simulink library "drf"  (Simulink 8.1)
settings: Solver=ode1  StartTime=0.0  StopTime=Inf  FixedStep=0.001  RelTol=1e-3
PostLoadFcn:
  | , if any(exist('dsrtsu_mdlpostloadfcn', 'file') == [2, 3, 6]), try dsrtsu_mdlpostloadfcn('Execute', bdroot); catch fprintf('Error in PostLoadFcn (dsrtsu_mdlpostloadfcn) for model "%s":\n %s\n', bdroot, lasterr); end, end,
undefined symbols (not defined in the file or in its folder): ZERO_FLOAT
libraries: drd x1, drg x1
settings Model: DSRTSU_INTERNAL_RTI_VER=450  DSRTSU_INTERNAL_RTI_TYPE=rti1401  RTICANMMDATA=struct('GeneralSetupData',struct('modelroot','D:\ELN150201_TAIWAN\trunk\AdasDragon\software\sw_development\arch\app\acc','generalsettings',struct('filesettings',struct('destfolder',struct('Name','RTICANMM_FILES','Check',1),'buildfolder',struct('Name','.','Check',1),'AbsDestfolder',struct('Name','D:\ELN150201_TAIWAN\trunk\AdasDragon\software\sw_development\arch\app\acc\RTICANMM_FILES'),'AbsBuildfolder',struct('Name','D:\ELN150201_TAIWAN\trunk\AdasDragon\software\sw_development\arch\app\acc'))),'options',struct('addpaths',1,'rmpaths',1,'addtrcexclusion',logical(1),'cannavigator',struct('checkmonitoring',0),'show_usrtrc',0,'use_usrtrc',0),'advanced',struct('options',[1 1 1 1 1 1 1 1 1 1 1 1 1 1 1 1 1 1 1 1 1 1 1 1 1 1 1 1 1 1 1 1 1 1 1 1 1 1 1 1 1 1 1 1 1 1 1 1 1 1 1 1 1 1 1 1 1 1 1 1 1 1 1 1 1 1 1 1 1 1 1 1 1 1 1 1 1 1 1 1 1 1 1 1 1 1 1 1 1 1 1 1 1 1 1 1 1 1 1 1]),'MPSetup',{{}},'modelname','drd','block','drd'))  DSRTSU_INTERNAL_RTIFPGA=40  Creator=AT015555  LastModifiedBy=AT015555

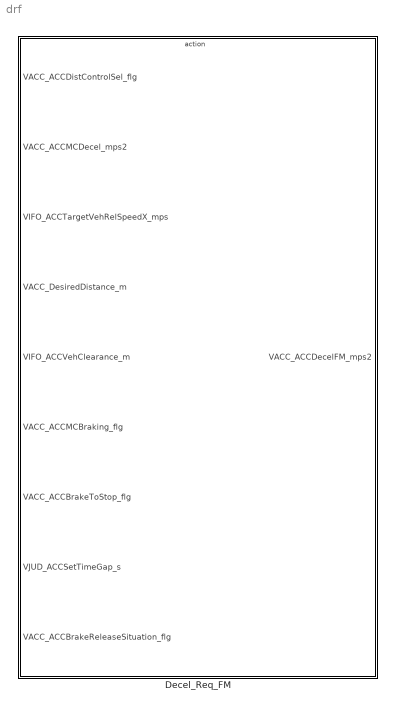
== system drf ==
  Decel_Req_FM : Subsystem  TreatAsAtomicUnit=on

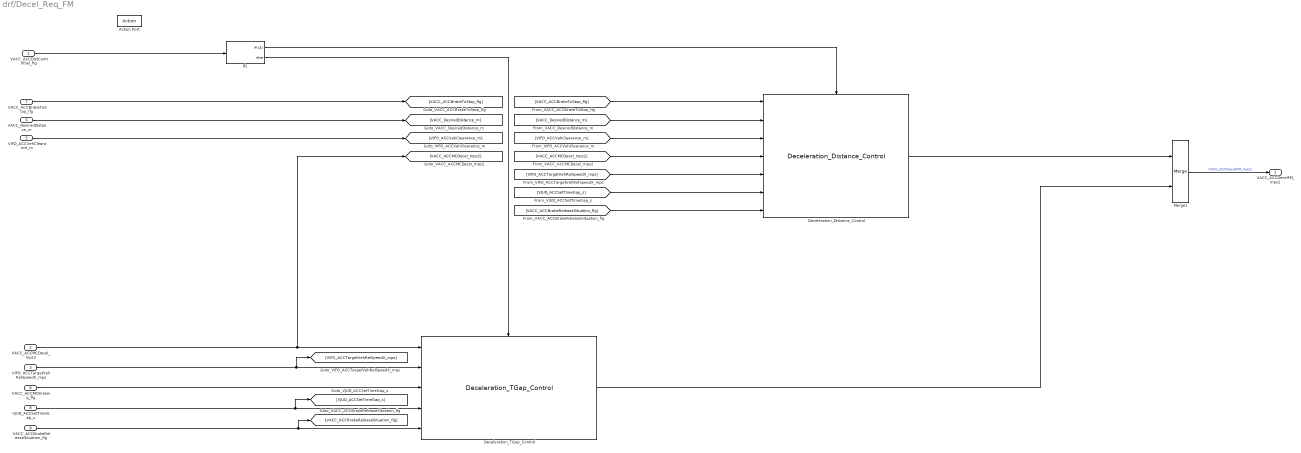
== system drf/Decel_Req_FM ==
  VACC_ACCDistControlSel_flg : Inport
  VACC_ACCMCDecel_mps2 : Inport  Port=2
  VIFO_ACCTargetVehRelSpeedX_mps : Inport  Port=3
  VACC_DesiredDistance_m : Inport  Port=4
  VIFO_ACCVehClearance_m : Inport  Port=5
  VACC_ACCMCBraking_flg : Inport  Port=6
  VACC_ACCBrakeToStop_flg : Inport  Port=7
  VJUD_ACCSetTimeGap_s : Inport  Port=8
  VACC_ACCBrakeReleaseSituation_flg : Inport  Port=9
  Action Port : ActionPort
  Deceleration_Distance_Control : drd/Deceleration_Distance_Control
  Deceleration_TGap_Control : drg/Deceleration_TGap_Control
  If2 : If  IfExpression=u1
  Merge1 : Merge
  VACC_ACCDecelFM_mps2 : Outport  OutputWhenDisabled=reset  InitialOutput=ZERO_FLOAT
  wires:
  VACC_ACCDistControlSel_flg/1 -> If2/1
  VACC_ACCMCDecel_mps2/1 -> Deceleration_TGap_Control/1, [VACC_ACCMCDecel_mps2]
  Merge1/1 -> VACC_ACCDecelFM_mps2/1  "VACC_ACCDecelFM_mps2"
  If2/2 -> Deceleration_TGap_Control/Action
  If2/1 -> Deceleration_Distance_Control/Action
  VIFO_ACCTargetVehRelSpeedX_mps/1 -> Deceleration_TGap_Control/2, [VIFO_ACCTargetVehRelSpeedX_mps]
  VACC_DesiredDistance_m/1 -> [VACC_DesiredDistance_m]
  [VACC_DesiredDistance_m] -> Deceleration_Distance_Control/2
  VIFO_ACCVehClearance_m/1 -> [VIFO_ACCVehClearance_m]
  [VIFO_ACCVehClearance_m] -> Deceleration_Distance_Control/3
  Deceleration_Distance_Control/1 -> Merge1/1
  Deceleration_TGap_Control/1 -> Merge1/2
  VACC_ACCMCBraking_flg/1 -> Deceleration_TGap_Control/3
  [VIFO_ACCTargetVehRelSpeedX_mps] -> Deceleration_Distance_Control/5
  [VACC_ACCMCDecel_mps2] -> Deceleration_Distance_Control/4
  VACC_ACCBrakeToStop_flg/1 -> [VACC_ACCBrakeToStop_flg]
  [VACC_ACCBrakeToStop_flg] -> Deceleration_Distance_Control/1
  VJUD_ACCSetTimeGap_s/1 -> Deceleration_TGap_Control/4, [VJUD_ACCSetTimeGap_s]
  [VJUD_ACCSetTimeGap_s] -> Deceleration_Distance_Control/6
  [VACC_ACCBrakeReleaseSituation_flg] -> Deceleration_Distance_Control/7
  VACC_ACCBrakeReleaseSituation_flg/1 -> Deceleration_TGap_Control/5, [VACC_ACCBrakeReleaseSituation_flg]
